simulink model "LEO_EMC_Sim_Simulink"  (R2021a)
settings: Solver=FixedStepDiscrete  StartTime=0.0  StopTime=cfg.sim.StopTime  FixedStep=cfg.sim.Ts  RelTol=1e-3
values from neighbouring files (symbols this model uses):
  cfg = defaultConfig()    [LEO_Sim_V1.m]    (also in build_LEO_EMC_Sim.m = evalin('base','cfg'); cfo_comp.m = evalin('base','cfg'); interf_gen.m = evalin('base','cfg'); preamble_insert.m = evalin('base','cfg'))
undefined symbols (not defined in the file or in its folder): doppler
libraries: commchan3 x2, commrandsrc3 x2, commdigbbndam3 x2, commcnvcod2 x2, commrflib2 x1
settings Model: Creator=52834  LastModifiedBy=52834

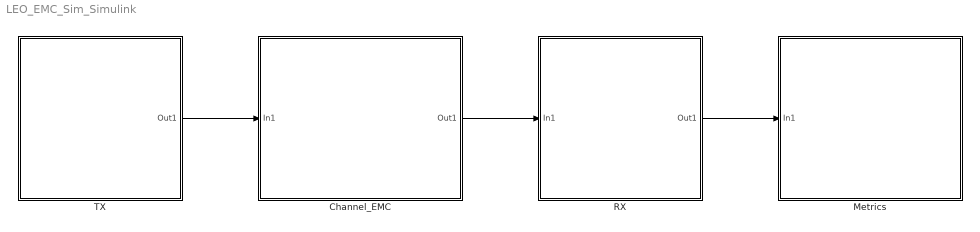
== system LEO_EMC_Sim_Simulink ==
  Channel_EMC : Subsystem
  Metrics : Subsystem
  RX : Subsystem
  TX : Subsystem
  wires:
  TX/1(Out1) -> Channel_EMC/1(In1)
  Channel_EMC/1(Out1) -> RX/1(In1)
  RX/1(Out1) -> Metrics/1(In1)

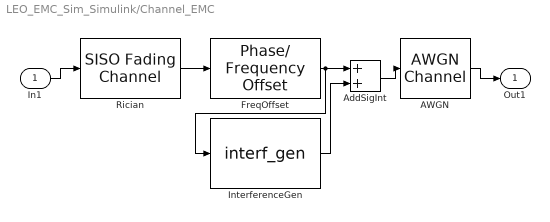
== system LEO_EMC_Sim_Simulink/Channel_EMC ==
  In1 : Inport
  AWGN : commchan3/AWGN Channel  InputProcessing=Columns as channels (frame based)  seed=67  noiseMode="Signal to noise ratio  (Eb/No)"  EbNodB=cfg.noise.EbN0_dB  EsNodB=10  SNRdB=10  bitsPerSym=2  Ps=1  Tsym=cfg.sim.Ts  variance=1
  AddSigInt : Sum
  FreqOffset : commrflib2/Phase// Frequency Offset  phaseOffset=0  freqPort=off  freqOffset=cfg.leo.fD_Hz
  InterferenceGen : MATLABFcn  MATLABFcn=interf_gen  OutputDimensions=1032
  Rician : commchan3/SISO Fading Channel  InheritSampleRate=on  SampleRate=1  PathDelays=0  AveragePathGains=0  NormalizePathGains=on  FadingDistribution=Rician  KFactor=10^(cfg.chan.K_dB/10)  DirectPathDopplerShift=0  DirectPathInitialPhase=0  MaximumDopplerShift=0  DopplerSpectrum=doppler('Jakes')  RandomStream=mt19937ar with seed  Seed=73  PathGainsOutputPort=off  ChannelFilterDelayOutputPort=off  SimulateUsing=Interpreted execution  Visualization=Off  PathsForDopplerDisplay=1  SamplesToDisplay=25%
  Out1 : Outport
  wires:
  In1/1 -> Rician/1
  Rician/1 -> FreqOffset/1
  FreqOffset/1 -> AddSigInt/1, InterferenceGen/1
  InterferenceGen/1 -> AddSigInt/2
  AddSigInt/1 -> AWGN/1
  AWGN/1 -> Out1/1

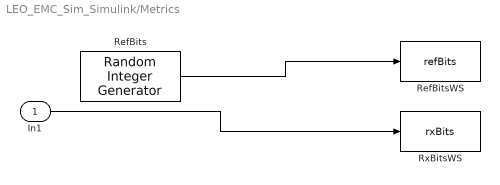
== system LEO_EMC_Sim_Simulink/Metrics ==
  In1 : Inport
  RefBits : commrandsrc3/Random Integer Generator  SetSize=2  SeedSource=Auto  Seed=0  SampleTime=cfg.sim.Ts * (cfg.phy.frameBits + cfg.phy.preambleHalfLen * cfg.phy.preambleReps)  SamplesPerFrame=cfg.phy.frameBits + cfg.phy.preambleHalfLen * cfg.phy.preambleReps  OutputDataType=double  SimulateUsing=Interpreted execution
  RefBitsWS : ToWorkspace  VariableName=refBits  SampleTime=-1
  RxBitsWS : ToWorkspace  VariableName=rxBits  SampleTime=-1
  wires:
  RefBits/1 -> RefBitsWS/1
  In1/1 -> RxBitsWS/1

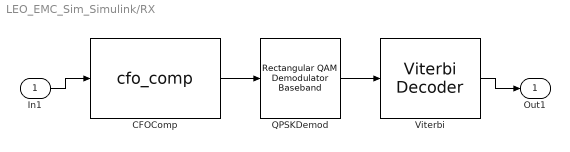
== system LEO_EMC_Sim_Simulink/RX ==
  In1 : Inport
  CFOComp : MATLABFcn  MATLABFcn=cfo_comp  OutputDimensions=1032
  QPSKDemod : commdigbbndam3/Rectangular QAM Demodulator Baseband  M=4  OutType=Bit  DecType=Hard decision  VarSource=Dialog  Variance=1  Dec=Gray  Mapping=[0:15]  PowType=Average Power  MinDist=2  AvgPow=1  PeakPow=1  Ph=0  outDtype1=Inherit via internal rule  outDtype2=Inherit via internal rule  derotateFactorWordLen=16  derotateFactorDataTypeStr=Inherit: Same word length as input  derotateFactorLastDataTypeStr=Inherit: Same word length as input  denormFactorWordLen=16  denormFactorDataTypeStr=Inherit: Same word length as input  denormFactorLastDataTypeStr=Inherit: Same word length as input  prodOutWordLen=32  prodOutOverflowMode=Wrap  prodOutRoundingMode=Floor  prodOutOvFlMode=off  prodOutOvFlModeLastStrValue=off  sumWordLen=32
  Viterbi : commcnvcod2/Viterbi Decoder  trellis=poly2trellis(7,[171 133])  isPunctured=off  punctureVector=[1; 1; 0; 1; 0; 1]  erasures=off  dectype=Hard decision  nsdecb=4  runSigValErrCheck=off  tbdepth=42  opmode=Terminated  reset=off  delayedResetAction=off  smWordLength=16  outDataType=Inherit via internal rule
      settings: SourceProductBaseCode=CM
  Out1 : Outport
  wires:
  In1/1 -> CFOComp/1
  CFOComp/1 -> QPSKDemod/1
  QPSKDemod/1 -> Viterbi/1
  Viterbi/1 -> Out1/1

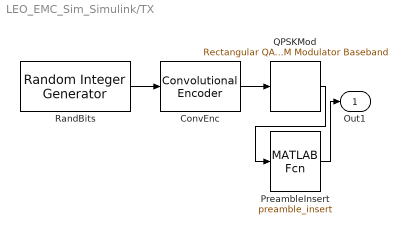
== system LEO_EMC_Sim_Simulink/TX ==
  ConvEnc : commcnvcod2/Convolutional Encoder  trellis=poly2trellis(7,[171 133])  opMode=Continuous  DelayedResetAction=off  hasIniStPort=off  hasFinStPort=off  usePuncVector=off  punctureVector=[1; 1; 0; 1; 0; 1]  reset=Unused parameter value
      settings: SourceProductBaseCode=CM
  PreambleInsert : MATLABFcn  MATLABFcn=preamble_insert  OutputDimensions=1032
  QPSKMod : commdigbbndam3/Rectangular QAM Modulator Baseband  M=4  InType=Bit  Enc=Gray  Mapping=[0:15]  PowType=Average Power  MinDist=2  AvgPow=1  PeakPow=1  Ph=0  outDtype=double  outWordLen=16  outUDDataType=sfix(16)  outFracLenMode=Best precision  outFracLen=15  outDataTypeStr=double  outLastDataTypeStr=double
  RandBits : commrandsrc3/Random Integer Generator  SetSize=2  SeedSource=Auto  Seed=0  SampleTime=cfg.sim.Ts  SamplesPerFrame=cfg.phy.frameBits  OutputDataType=double  SimulateUsing=Interpreted execution
  Out1 : Outport
  wires:
  RandBits/1 -> ConvEnc/1
  ConvEnc/1 -> QPSKMod/1
  QPSKMod/1 -> PreambleInsert/1
  PreambleInsert/1 -> Out1/1
